simulink model "Simulation"  (R2018b)
settings: Solver=VariableStepAuto  StartTime=0.0  StopTime=tmax  RelTol=1e-3
values from neighbouring files (symbols this model uses):
  i = i+1    (= 2)    [PowerRegen.m]    (also in RunSimulation.m = -0.005; RunSimulationKF.m = -0.005)
  mL = 650    [PowerRegen.m]    (also in RunSimulation.m; RunSimulationKF.m)
  mWz = 1200    [RunSimulation.m]    (also in RunSimulationKF.m)
  Pres = 1/1000*[5.7/771 0 1.6]    [RunSimulation.m]    (also in RunSimulationKF.m)
  s0 = 0    [RunSimulation.m]    (also in RunSimulationKF.m)
  Ts = sysd.Ts    [RunSimulation.m]    (also in RunSimulationKF.m = 0.015)
  v0 = 10/3.6    (= 2.77777777778)    [RunSimulation.m]    (also in RunSimulationKF.m = 3.33333333333)
undefined symbols (not defined in the file or in its folder): Discrete, Time
libraries: ctrlSharedLib x1
settings Model: Creator=raphael  LastModifiedBy=raphael

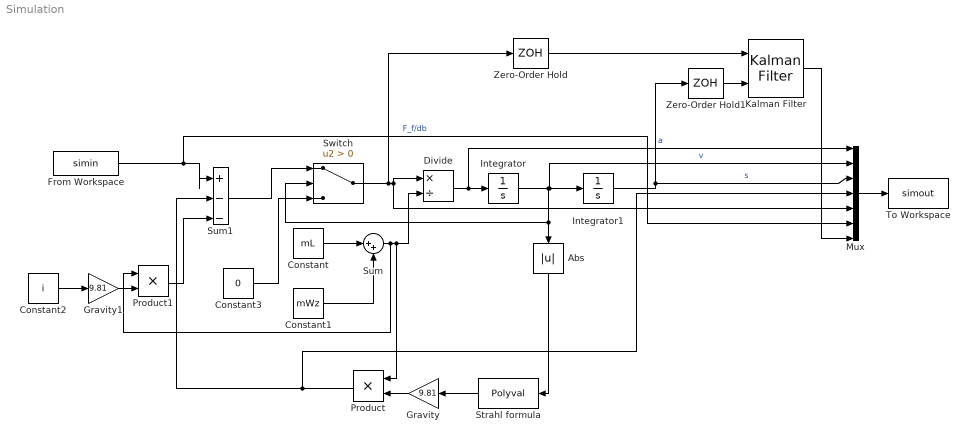
== system Simulation ==
  Abs : Abs
  Constant : Constant  Value=mL
  Constant1 : Constant  Value=mWz
  Constant2 : Constant  Value=i
  Constant3 : Constant  Value=0
  Divide : Product  Inputs=*/
  From Workspace : FromWorkspace  VariableName=simin  SampleTime=0
  Gravity : Gain  Gain=9.81
  Gravity1 : Gain  Gain=9.81
  Integrator : Integrator  InitialCondition=v0
  Integrator1 : Integrator  InitialCondition=s0
  Kalman Filter : ctrlSharedLib/Kalman Filter  TimeDomain=Discrete-Time  UseCurrentEstimator=off  ModelSource=LTI State-Space Variable  ModelSourceVariable=sysSS  A=0.95*eye(2)  B=eye(2)  C=eye(2)  D=zeros(2)  NumberOfStates=2  NumberOfInputs=2  NumberOfOutputs=2  InitialEstimateSource=Dialog  X0=0  P0=10  UseK=off  UseGH=off  NumberOfProcessNoiseInputs=2  G=1  TimeInvariantG=on  H=0  TimeInvariantH=on  Q=0.05  TimeInvariantQ=on  R=1  TimeInvariantR=on  N=0  TimeInvariantN=on  AddInputPort=on  AddEnablePort=off  OutputEstimatedY=off  OutputP=off  Ts=-1
      settings: SourceProductBaseCode=CT
  Mux : Mux  Inputs=7
  Product : Product
  Product1 : Product
  Strahl formula : Polyval  Coefs=Pres
  Sum : Sum  Inputs=|++
  Sum1 : Sum  Inputs=|+--
  Switch : Switch  Criteria=u2 > Threshold
  To Workspace : ToWorkspace  VariableName=simout  SaveFormat=Timeseries  SampleTime=-1
  Zero-Order Hold : ZeroOrderHold  SampleTime=Ts
  Zero-Order Hold1 : ZeroOrderHold  SampleTime=Ts
  wires:
  Constant/1 -> Sum/1
  Constant1/1 -> Sum/2
  Sum/1 -> Product1/1, Product/1, Divide/2
  Divide/1 -> Mux/1, Integrator/1  "a"
  Integrator/1 -> Mux/2, Integrator1/1, Switch/2, Abs/1  "v"
  From Workspace/1 -> Mux/6, Sum1/1  "F_f/db"
  Gravity/1 -> Product/2
  Strahl formula/1 -> Gravity/1
  Product/1 -> Mux/4, Sum1/2
  Constant2/1 -> Gravity1/1
  Gravity1/1 -> Product1/2
  Product1/1 -> Sum1/3
  Integrator1/1 -> Zero-Order Hold1/1, Mux/3  "s"
  Mux/1 -> To Workspace/1
  Abs/1 -> Strahl formula/1
  Switch/1 -> Zero-Order Hold/1, Divide/1, Mux/5
  Sum1/1 -> Switch/1
  Constant3/1 -> Switch/3
  Zero-Order Hold/1 -> Kalman Filter/1
  Zero-Order Hold1/1 -> Kalman Filter/2
  Kalman Filter/1 -> Mux/7
